simulink model "inverted_pendulum_fuzzy_control"  (R2021b)
settings: Solver=VariableStepAuto  StartTime=0.0  StopTime=10.0  RelTol=1e-3
libraries: fuzblock x1
settings Model: Creator=william  LastModifiedBy=william

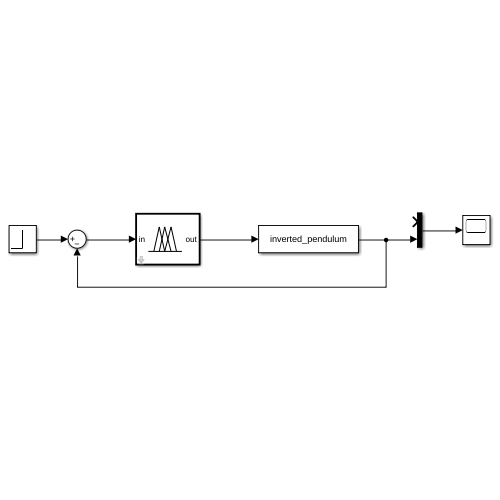
[thumbnail: Simulink's stored preview of the top-level diagram]
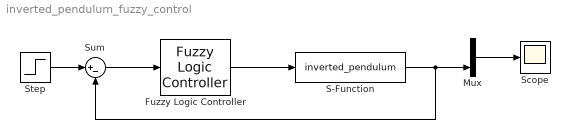
== system inverted_pendulum_fuzzy_control ==
  Fuzzy Logic Controller : fuzblock/Fuzzy Logic  Controller  FIS='tipper.fis'  OutputSampleNumber=101  DataType=double  FuzzifiedInputs=off  RuleFiringStrengths=off  RuleOutputs=off  AggregatedOutputs=off  SimulateUsing=Interpreted execution  OutOfRangeInputValueMessage=warning  NoRuleFiredMessage=warning  EmptyOutputFuzzySetMessage=warning
  Mux : Mux  Inputs=2
  S-Function : S-Function  FunctionName=inverted_pendulum  SFunctionDeploymentMode=off  EnableBusSupport=off
  Scope : Scope
  Step : Step  Time=0  After=0  SampleTime=0
  Sum : Sum  Inputs=|+-
  wires:
  Fuzzy Logic Controller/1 -> S-Function/1
  S-Function/1 -> Sum/2, Mux/2
  Mux/1 -> Scope/1
  Sum/1 -> Fuzzy Logic Controller/1
  Step/1 -> Sum/1
